simulink model "SistemaGrua_Planta_ModeloCompleto"  (R2020b)
settings: Solver=ode45  StartTime=0.0  StopTime=10  FixedStep=1e-3  RelTol=1e-3
values from neighbouring files (symbols this model uses):
  bcx = 1e6    (= 1000000)    [Valores_1.m]    (also in valoresPlanta.m; valoresPlanta_29_9_24.m; valoresPlanta_V3.m; valoresPlanta_v4.m)
  bcy = 1e7    (= 10000000)    [Valores_1.m]    (also in valoresPlanta.m; valoresPlanta_29_9_24.m; valoresPlanta_V3.m; valoresPlanta_v4.m)
  beq = bt+(btd+btm*it^2)/rtd^2    (= 21697.2)    [Valores.m]    (also in Valores_1.m; valoresPlanta_29_9_24.m; valoresPlanta_v4.m)
  bh_eq = bhm*ih^2+bhd    (= 8720)    [Valores.m]    (also in Valores_1.m; valoresPlanta.m; valoresPlanta_29_9_24.m; valoresPlanta_V3.m)
  bhb = 1e8    (= 100000000)    [Valores.m]    (also in Valores_1.m; valoresPlanta.m; valoresPlanta_29_9_24.m; valoresPlanta_V3.m)
  bhEb = 2.2e9    (= 2200000000)    [Valores.m]    (also in Valores_1.m; valoresPlanta.m; valoresPlanta_29_9_24.m; valoresPlanta_V3.m)
  bt = 90.0    (= 90)    [Valores.m]    (also in Valores_1.m; valoresPlanta.m; valoresPlanta_29_9_24.m; valoresPlanta_V3.m)
  btm = 6.0    (= 6)    [Valores.m]    (also in Valores_1.m; valoresPlanta.m; valoresPlanta_29_9_24.m; valoresPlanta_V3.m)
  btw = 3.0e3    (= 3000)    [Valores.m]    (also in Valores_1.m; valoresPlanta.m; valoresPlanta_29_9_24.m; valoresPlanta_V3.m)
  bwu = 150    [Valores.m]    (also in Valores_1.m; valoresPlanta.m; valoresPlanta_29_9_24.m; valoresPlanta_V3.m)
  g = 9.80665    [Valores.m]    (also in Valores_1.m; valoresPlanta.m; valoresPlanta_29_9_24.m; valoresPlanta_V3.m)
  ih = 22    [Valores.m]    (also in Valores_1.m; valoresPlanta.m; valoresPlanta_29_9_24.m; valoresPlanta_V3.m)
  it = 30    [Valores.m]    (also in Valores_1.m; valoresPlanta.m; valoresPlanta_29_9_24.m; valoresPlanta_V3.m)
  Jh_eq = Jhm_hb*ih^2+Jhd_hEb    (= 18320)    [Valores.m]    (also in Valores_1.m; valoresPlanta.m; valoresPlanta_29_9_24.m; valoresPlanta_V3.m)
  Jtm_tb = 7.0    (= 7)    [Valores.m]    (also in Valores_1.m; valoresPlanta.m; valoresPlanta_29_9_24.m; valoresPlanta_V3.m)
  kcy = 1.8e9    (= 1800000000)    [Valores_1.m]    (also in valoresPlanta.m; valoresPlanta_29_9_24.m; valoresPlanta_V3.m; valoresPlanta_v4.m)
  KDh = Jeq2 * w_posh^3    (= -12245.4404091)    [Valores.m]    (also in Valores_1.m = Jeq2 * w_posh; valoresPlanta.m = Jeq2 * w_posh; valoresPlanta_29_9_24.m = Jh_eq * n * w_posh; valoresPlanta_V3.m = Jeq2 * w_posh)
  KDt = Meq2 * w_post^3    (= -4728.86946035)    [Valores.m]    (also in Valores_1.m = Meq2 * w_post; valoresPlanta.m = Meq2 * w_post; valoresPlanta_29_9_24.m = 10127; valoresPlanta_V3.m = Meq2 * w_post)
  KIh = Jeq2 * w_posh^2    (= 2572.66592082)    [Valores.m]    (also in Valores_1.m = Jeq2 * w_posh^3; valoresPlanta.m = Jeq2 * w_posh^3; valoresPlanta_29_9_24.m = Jh_eq * w_posh^3; valoresPlanta_V3.m = Jeq2 * w_posh^3)
  KIt = Meq2 * w_post^2    (= 1307.690244)    [Valores.m]    (also in Valores_1.m = Meq2 * w_post^3; valoresPlanta.m = Meq2 * w_post^3; valoresPlanta_29_9_24.m = 6809.6; valoresPlanta_V3.m = Meq2 * w_post^3)
  KPh = Jeq2 * w_posh    (= -540.495867769)    [Valores.m]    (also in Valores_1.m = Jeq2 * w_posh^2; valoresPlanta.m = Jeq2 * w_posh^2; valoresPlanta_29_9_24.m = Jh_eq * n * w_posh^2; valoresPlanta_V3.m = Jeq2 * w_posh^2)
  KPt = Meq2 * w_post    (= -361.62)    [Valores.m]    (also in Valores_1.m = Meq2 * w_post^2; valoresPlanta.m = Meq2 * w_post^2; valoresPlanta_29_9_24.m = 14123; valoresPlanta_V3.m = Meq2 * w_post^2)
  Ktw = 4.8e5    (= 480000)    [Valores.m]    (also in Valores_1.m; valoresPlanta.m; valoresPlanta_29_9_24.m; valoresPlanta_V3.m)
  kwu = 2.36e8    (= 236000000)    [Valores.m]    (also in Valores_1.m; valoresPlanta.m; valoresPlanta_29_9_24.m; valoresPlanta_V3.m)
  Mc_max = 5e4    (= 50000)    [Valores.m]    (also in Valores_1.m; valoresPlanta.m; valoresPlanta_29_9_24.m; valoresPlanta_V3.m)
  Mc_min = 2e3    (= 2000)    [Valores.m]    (also in Valores_1.m; valoresPlanta.m; valoresPlanta_29_9_24.m; valoresPlanta_V3.m)
  Meq = Mt+(it^2*Jtm_tb+Jtd)/rtd^2    (= 60000)    [Valores.m]    (also in Valores_1.m; valoresPlanta_29_9_24.m; valoresPlanta_v4.m)
  Ms = 1.5e4    (= 15000)    [Valores.m]    (also in Valores_1.m; valoresPlanta.m; valoresPlanta_29_9_24.m; valoresPlanta_V3.m)
  Mt = 30000    [Valores.m]    (also in Valores_1.m; valoresPlanta.m; valoresPlanta_29_9_24.m; valoresPlanta_V3.m)
  rhd = 0.75    [Valores.m]    (also in Valores_1.m; valoresPlanta.m; valoresPlanta_29_9_24.m; valoresPlanta_V3.m)
  rtd = 0.5    [Valores.m]    (also in Valores_1.m; valoresPlanta.m; valoresPlanta_29_9_24.m; valoresPlanta_V3.m)
  tau_tm = 1e-3    (= 0.001)    [Valores.m]    (also in Valores_1.m; valoresPlanta.m; valoresPlanta_29_9_24.m; valoresPlanta_V3.m)
  tauhm = 1e-3    (= 0.001)    [Valores.m]    (also in Valores_1.m)
  Thb_Max = 5e4    (= 50000)    [Valores.m]    (also in Valores_1.m; valoresPlanta.m; valoresPlanta_29_9_24.m; valoresPlanta_V3.m)
  ThEb_Max = 1.1e6    (= 1100000)    [Valores.m]    (also in Valores_1.m; valoresPlanta.m; valoresPlanta_29_9_24.m; valoresPlanta_V3.m)
  Thm_Max = 2e4    (= 20000)    [Valores.m]    (also in Valores_1.m; valoresPlanta.m; valoresPlanta_29_9_24.m; valoresPlanta_V3.m)
  Ttb_Max = 5e3    (= 5000)    [Valores.m]    (also in Valores_1.m; valoresPlanta.m; valoresPlanta_29_9_24.m; valoresPlanta_V3.m)
  Ttm_Max = 3e3    (= 3000)    [Valores.m]    (also in Valores_1.m; valoresPlanta.m; valoresPlanta_29_9_24.m = 4000; valoresPlanta_V3.m)
  Yt0 = 45    [Valores.m]    (also in Valores_1.m; valoresPlanta.m; valoresPlanta_29_9_24.m; valoresPlanta_V3.m)
undefined symbols (not defined in the file or in its folder): DiscIntNeverNeededParam, sigbuilder_block
libraries: simulink x1, simulink_extras x1
settings Model: Creator=Matias  LastModifiedBy=agustin

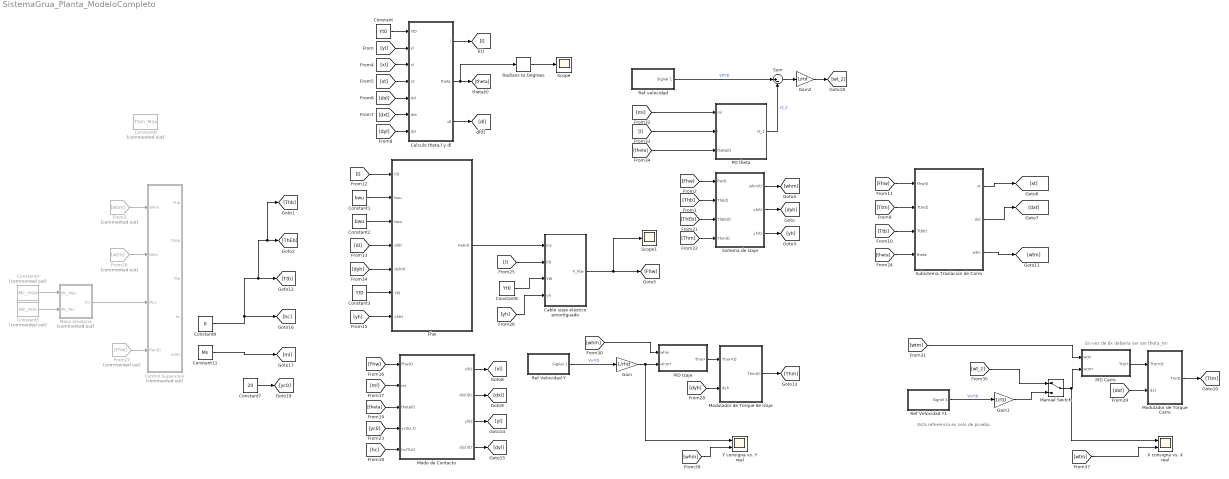
== system SistemaGrua_Planta_ModeloCompleto ==
  note: Esta referencia es solo de prueba
  note: En vez de dx debería ser ser theta_tm
  Cable izaje elástico amortiguado : Subsystem
  Calculo theta,l y dl : Subsystem
  Constant : Constant  Value=Yt0
  Constant1 : Constant  Value=kwu
  Constant11 : Constant  Value=Ms
  Constant2 : Constant  Value=bwu
  Constant3 : Constant  Value=Yt0
  Constant4 : Constant  Commented=on  Value=Mc_max
  Constant5 : Constant  Commented=on  Value=Mc_min
  Constant6 : Constant  Commented=on  Value=Thm_Max
  Constant7 : Constant  Value=20
  Constant8 : Constant  Value=Yt0
  Constant9 : Constant  Value=0
  Control Supervisor : Subsystem  Commented=on
  Fhw : Subsystem
  From20 : From  Commented=on  GotoTag=wtm
  From27 : From  Commented=on  GotoTag=Fhw
  From3 : From  Commented=on  GotoTag=whm
  Gain : Gain  Gain=1/rhd
  Gain1 : Gain  Gain=1/rtd
  Gain2 : Gain  Gain=1/rtd
  Manual Switch : ManualSwitch
  Masa aleatoria : MATLAB Function  Commented=on  TreatAsAtomicUnit=on
  Modo de Contacto : Subsystem
  Modulador de Torque Carro : Subsystem
  Modulador de Torque de Izaje : Subsystem
  PD theta : Subsystem
  PID Carro : Subsystem
  PID Izaje : Subsystem
  Radians to Degrees : simulink_extras/Transformations/Radians to Degrees
  Ref Velocidad Y : Subsystem  Tag=STV Subsys  LoadFcn=sigbuilder_block('load');  StartFcn=sigbuilder_block('start');  StopFcn=sigbuilder_block('stop');  ClipboardFcn=sigbuilder_block('clipboard');  mask(Sigbuilder block){tuvar=[0:10]}
      mask help: Simulink:masks:SigbuilderBlock_MD
      mask init:
      | if ~strcmp(get_param(bdroot(gcbh),'SimulationStatus'),'stopped') tuvar = sigbuilder_block('maskInit'); end
      settings: CopyFcn=sigbuilder_block('copy');  DeleteFcn=sigbuilder_block('delete');  ModelCloseFcn=sigbuilder_block('modelClose');  PreSaveFcn=sigbuilder_block('preSave');  PauseFcn=sigbuilder_block('pause');  ContinueFcn=sigbuilder_block('continue');  NameChangeFcn=sigbuilder_block('namechange');  OpenFcn=sigbuilder_block('open',[6 36 1012.5 476.25 ]);  CloseFcn=sigbuilder_block('close');
      mask Display: plot(0, 0, 100, 100,[2, 2, 32, 32, 2], [68, 8, 8, 68, 68],[32, 2], [38, 38], [32, 19, 2],[53, 60, 44], [32, 17, 17, 2],[16, 16, 31, 31]);txt = getActiveGroup(gcbh);text(2, 100, txt,'verticalAlignment', 'top');
  Ref Velocidad Y1 : Subsystem  Tag=STV Subsys  LoadFcn=sigbuilder_block('load');  StartFcn=sigbuilder_block('start');  StopFcn=sigbuilder_block('stop');  ClipboardFcn=sigbuilder_block('clipboard');  mask(Sigbuilder block){tuvar=[0:10]}
      mask help: Simulink:masks:SigbuilderBlock_MD
      mask init:
      | if ~strcmp(get_param(bdroot(gcbh),'SimulationStatus'),'stopped') tuvar = sigbuilder_block('maskInit'); end
      settings: CopyFcn=sigbuilder_block('copy');  DeleteFcn=sigbuilder_block('delete');  ModelCloseFcn=sigbuilder_block('modelClose');  PreSaveFcn=sigbuilder_block('preSave');  PauseFcn=sigbuilder_block('pause');  ContinueFcn=sigbuilder_block('continue');  NameChangeFcn=sigbuilder_block('namechange');  OpenFcn=sigbuilder_block('open',[6 30 1012.5 447.75 ]);  CloseFcn=sigbuilder_block('close');
      mask Display: plot(0, 0, 100, 100,[2, 2, 32, 32, 2], [68, 8, 8, 68, 68],[32, 2], [38, 38], [32, 19, 2],[53, 60, 44], [32, 17, 17, 2],[16, 16, 31, 31]);txt = getActiveGroup(gcbh);text(2, 100, txt,'verticalAlignment', 'top');
  Ref velocidad : Subsystem  Tag=STV Subsys  LoadFcn=sigbuilder_block('load');  StartFcn=sigbuilder_block('start');  StopFcn=sigbuilder_block('stop');  ClipboardFcn=sigbuilder_block('clipboard');  mask(Sigbuilder block){tuvar=[0:10]}
      mask help: Simulink:masks:SigbuilderBlock_MD
      mask init:
      | if ~strcmp(get_param(bdroot(gcbh),'SimulationStatus'),'stopped') tuvar = sigbuilder_block('maskInit'); end
      settings: CopyFcn=sigbuilder_block('copy');  DeleteFcn=sigbuilder_block('delete');  ModelCloseFcn=sigbuilder_block('modelClose');  PreSaveFcn=sigbuilder_block('preSave');  PauseFcn=sigbuilder_block('pause');  ContinueFcn=sigbuilder_block('continue');  NameChangeFcn=sigbuilder_block('namechange');  OpenFcn=sigbuilder_block('open',[6 36 1012.5 476.25 ]);  CloseFcn=sigbuilder_block('close');
      mask Display: plot(0, 0, 100, 100,[2, 2, 32, 32, 2], [68, 8, 8, 68, 68],[32, 2], [38, 38], [32, 19, 2],[53, 60, 44], [32, 17, 17, 2],[16, 16, 31, 31]);txt = getActiveGroup(gcbh);text(2, 100, txt,'verticalAlignment', 'top');
  Scope : Scope
  Scope1 : Scope
  Sistema de Izaje : Subsystem
  Subsitema Traslación de Carro : Subsystem
  Sum : Sum  Inputs=|+-
  X consigna vs. X real : Scope  NumInputPorts=2
  Y consigna vs. Y real : Scope  NumInputPorts=2
  wires:
  From3/1 -> Control Supervisor/1(Whm)
  [Thb] -> Sistema de Izaje/2(Thb(t))
  [Fhw] -> Sistema de Izaje/1(Fw(t))
  Calculo theta,l y dl/1(l) -> [l]
  Calculo theta,l y dl/2(theta) -> [theta], Radians to Degrees/1
  Constant/1 -> Calculo theta,l y dl/1(Yt0)
  [xt] -> Calculo theta,l y dl/4(xt)
  [xl] -> Calculo theta,l y dl/3(xl)
  [yl] -> Calculo theta,l y dl/2(yl)
  Calculo theta,l y dl/3(dl) -> [dl]
  [dyl] -> Calculo theta,l y dl/7(dyl)
  [dxt] -> Calculo theta,l y dl/6(dxt)
  [dxl] -> Calculo theta,l y dl/5(dxl)
  [yh] -> Fhw/7(yh(t))
  [dyh] -> Fhw/5(dyh(t))
  [dl] -> Fhw/4(dl(t))
  [l] -> Fhw/1(l(t))
  Constant1/1 -> Fhw/2(kwu)
  Constant2/1 -> Fhw/3(bwu)
  [Ttb] -> Subsitema Traslación de Carro/3(Ttb(t))
  [Fhw] -> Subsitema Traslación de Carro/1(Fhw(t))
  [Ttm] -> Subsitema Traslación de Carro/2(Ttm(t))
  Subsitema Traslación de Carro/1(xt) -> [xt]
  Subsitema Traslación de Carro/2(dxt) -> [dxt]
  Modulador de Torque Carro/1(Tm(t)) -> [Ttm]
  Subsitema Traslación de Carro/3(wtm) -> [wtm]
  From20/1 -> Control Supervisor/2(Wtm)
  Modulador de Torque de Izaje/1(Thm(t)) -> [Thm]
  Sistema de Izaje/1(whm(t)) -> [whm]
  Sistema de Izaje/2(vh(t)) -> [dyh]
  Sistema de Izaje/3(yh(t)) -> [yh]
  [ThEb] -> Sistema de Izaje/3(ThEb(t))
  [Thm] -> Sistema de Izaje/4(Thm(t))
  Constant3/1 -> Fhw/6(Yt0)
  Constant5/1 -> Masa aleatoria/2(Mc_Min)
  Constant4/1 -> Masa aleatoria/1(Mc_Max)
  Masa aleatoria/1(ml) -> Control Supervisor/3(Mcx)
  [theta] -> Subsitema Traslación de Carro/4(theta)
  [yc0] -> Modo de Contacto/4(yc0(x,t))
  Modo de Contacto/2(d(xl)(t)) -> [dxl]
  Modo de Contacto/1(xl(t)) -> [xl]
  [hc] -> Modo de Contacto/5(hc(TLK))
  Modo de Contacto/4(d(yl)(t)) -> [dyl]
  [theta] -> Modo de Contacto/3(theta(t))
  Modo de Contacto/3(yl(t)) -> [yl]
  [ml] -> Modo de Contacto/2(ml)
  [Fhw] -> Modo de Contacto/1(Fhw(t))
  Fhw/1(Fwh(t)) -> Cable izaje elástico amortiguado/1(In1)
  [l] -> Cable izaje elástico amortiguado/2(l(t))
  Constant8/1 -> Cable izaje elástico amortiguado/3(Yt0)
  [yh] -> Cable izaje elástico amortiguado/4(yh)
  From27/1 -> Control Supervisor/4(Fwh(t))
  [dyh] -> Modulador de Torque de Izaje/2(dyh)
  [dxt] -> Modulador de Torque Carro/2(dxt)
  PID Carro/1(Ttm*) -> Modulador de Torque Carro/1(Ttm*(t)')
  PID Izaje/1(Thm*) -> Modulador de Torque de Izaje/1(Thm*(t)')
  [wtm] -> PID Carro/1(wtm)
  [whm] -> PID Izaje/1(whm)
  Ref Velocidad Y/1(Signal 1) -> Gain/1  "Vy*(t)"
  [wt_2] -> Manual Switch/1
  [whm] -> Y consigna vs. Y real/2
  [wtm] -> X consigna vs. X real/2
  Ref velocidad/1(Signal 1) -> Sum/1  "Vt*(t)"
  Sum/1 -> Gain2/1
  Gain2/1 -> [wt_2]
  Manual Switch/1 -> X consigna vs. X real/1, PID Carro/2(wtm*)
  Ref Velocidad Y1/1(Signal 1) -> Gain1/1  "Vx*(t)"
  Gain1/1 -> Manual Switch/2
  Gain/1 -> Y consigna vs. Y real/1, PID Izaje/2(whm*)
  [theta] -> PD theta/3(theta(t))
  [l] -> PD theta/2(l)
  PD theta/1(xt_2) -> Sum/2  "xt_2"
  [ml] -> PD theta/1(ml)
  Cable izaje elástico amortiguado/1(F_htw) -> Scope1/1, [Fhw]
  Constant7/1 -> [yc0]
  Constant11/1 -> [ml]
  Constant9/1 -> [Thb], [ThEb], [Ttb], [hc]
  Radians to Degrees/1 -> Scope/1

== system SistemaGrua_Planta_ModeloCompleto/Cable izaje elástico amortiguado ==
  note: l_h
  In1 : Inport
  l(t) : Inport  Port=2
  Yt0 : Inport  Port=3
  yh : Inport  Port=4
  Constant9 : Constant  Value=0
  Relational Operator : RelationalOperator  OutDataTypeStr=boolean  RndMeth=Simplest
  Sum : Sum  Inputs=|++
  Switch1 : Switch  Criteria=u2 > Threshold
  F_htw : Outport
  wires:
  l(t)/1 -> Relational Operator/1
  Sum/1 -> Relational Operator/2
  In1/1 -> Switch1/1
  Yt0/1 -> Sum/1
  Constant9/1 -> Switch1/3
  Relational Operator/1 -> Switch1/2
  yh/1 -> Sum/2
  Switch1/1 -> F_htw/1

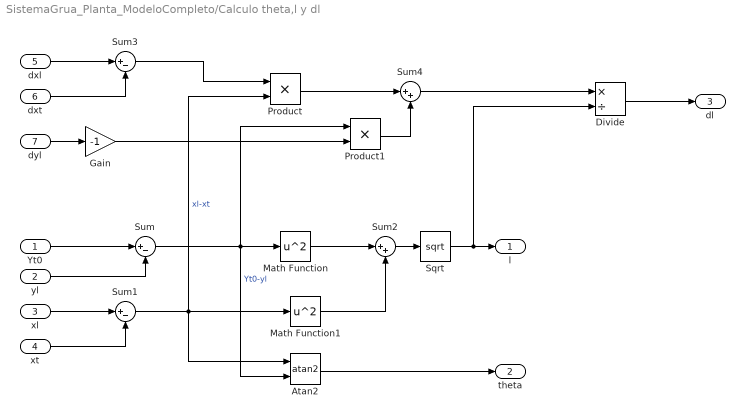
== system SistemaGrua_Planta_ModeloCompleto/Calculo theta,l y dl ==
  Yt0 : Inport
  yl : Inport  Port=2
  xl : Inport  Port=3
  xt : Inport  Port=4
  dxl : Inport  Port=5
  dxt : Inport  Port=6
  dyl : Inport  Port=7
  Atan2 : Trigonometry  Operator=atan2
  Divide : Product  Inputs=*/
  Gain : Gain  Gain=-1
  Math Function : Math  Operator=square  SaturateOnIntegerOverflow=on
  Math Function1 : Math  Operator=square  SaturateOnIntegerOverflow=on
  Product : Product
  Product1 : Product
  Sqrt : Sqrt  SaturateOnIntegerOverflow=on
  Sum : Sum  Inputs=|+-
  Sum1 : Sum  Inputs=|+-
  Sum2 : Sum  Inputs=|++
  Sum3 : Sum  Inputs=|+-
  Sum4 : Sum  Inputs=|++
  l : Outport
  theta : Outport  Port=2
  dl : Outport  Port=3
  wires:
  Yt0/1 -> Sum/1
  yl/1 -> Sum/2
  xl/1 -> Sum1/1
  xt/1 -> Sum1/2
  Atan2/1 -> theta/1
  Sum1/1 -> Product/2, Math Function1/1, Atan2/1  "xl-xt"
  Sum/1 -> Product1/1, Atan2/2, Math Function/1  "Yt0-yl"
  Math Function/1 -> Sum2/1
  Math Function1/1 -> Sum2/2
  Sum2/1 -> Sqrt/1
  Sqrt/1 -> Divide/2, l/1
  dxl/1 -> Sum3/1
  dxt/1 -> Sum3/2
  Sum3/1 -> Product/1
  dyl/1 -> Gain/1
  Gain/1 -> Product1/2
  Product/1 -> Sum4/1
  Product1/1 -> Sum4/2
  Sum4/1 -> Divide/1
  Divide/1 -> dl/1

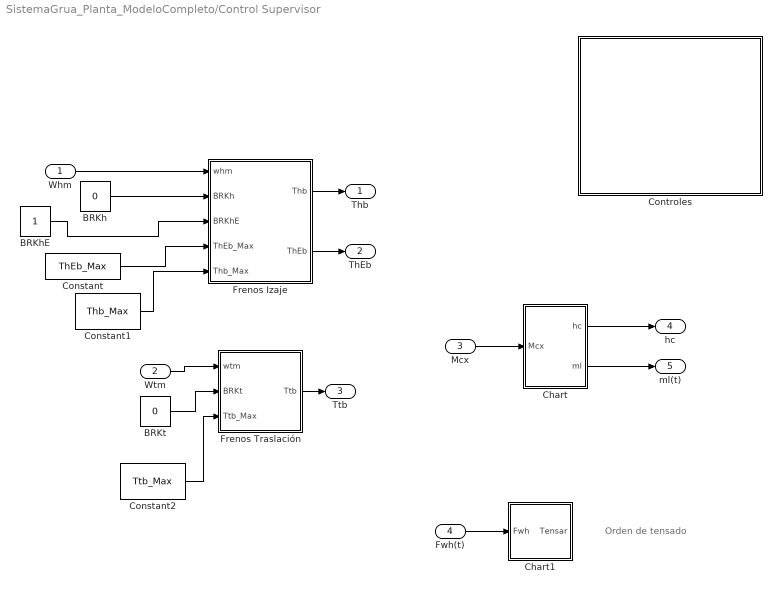
== system SistemaGrua_Planta_ModeloCompleto/Control Supervisor ==
  note: Orden de tensado
  Whm : Inport
  Wtm : Inport  Port=2
  Mcx : Inport  Port=3
  Fwh(t) : Inport  Port=4
  BRKh : Constant  Value=0
  BRKhE : Constant
  BRKt : Constant  Value=0
  Chart : Stateflow chart  TreatAsAtomicUnit=on
  Chart1 : Stateflow chart  TreatAsAtomicUnit=on
  Constant : Constant  Value=ThEb_Max
  Constant1 : Constant  Value=Thb_Max
  Constant2 : Constant  Value=Ttb_Max
  Controles : Subsystem
  "Frenos Izaje " : Stateflow chart  TreatAsAtomicUnit=on
  Frenos Traslación : Stateflow chart  TreatAsAtomicUnit=on
  Thb : Outport
  ThEb : Outport  Port=2
  Ttb : Outport  Port=3
  hc : Outport  Port=4
  ml(t) : Outport  Port=5
  wires:
  "Frenos Izaje "/1(Thb) -> Thb/1
  BRKh/1 -> "Frenos Izaje "/2(BRKh)
  Whm/1 -> "Frenos Izaje "/1(whm)
  BRKhE/1 -> "Frenos Izaje "/3(BRKhE)
  "Frenos Izaje "/2(ThEb) -> ThEb/1
  Wtm/1 -> Frenos Traslación/1(wtm)
  Frenos Traslación/1(Ttb) -> Ttb/1
  BRKt/1 -> Frenos Traslación/2(BRKt)
  Chart/2(ml) -> ml(t)/1
  Chart/1(hc) -> hc/1
  Mcx/1 -> Chart/1(Mcx)
  Fwh(t)/1 -> Chart1/1(Fwh)
  Constant/1 -> "Frenos Izaje "/4(ThEb_Max)
  Constant1/1 -> "Frenos Izaje "/5(Thb_Max)
  Constant2/1 -> Frenos Traslación/3(Ttb_Max)

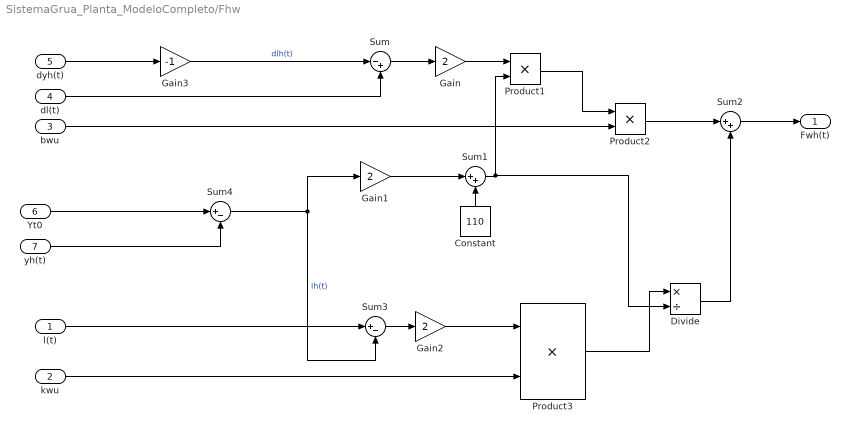
== system SistemaGrua_Planta_ModeloCompleto/Fhw ==
  l(t) : Inport
  kwu : Inport  Port=2
  bwu : Inport  Port=3
  dl(t) : Inport  Port=4
  dyh(t) : Inport  Port=5
  Yt0 : Inport  Port=6
  yh(t) : Inport  Port=7
  Constant : Constant  Value=110
  Divide : Product  Inputs=*/
  Gain : Gain  Gain=2
  Gain1 : Gain  Gain=2
  Gain2 : Gain  Gain=2
  Gain3 : Gain  Gain=-1
  Product1 : Product
  Product2 : Product
  Product3 : Product
  Sum : Sum  Inputs=|-+
  Sum1 : Sum  Inputs=|++
  Sum2 : Sum  Inputs=|++
  Sum3 : Sum  Inputs=|+-
  Sum4 : Sum  Inputs=|+-
  Fwh(t) : Outport
  wires:
  dl(t)/1 -> Sum/2
  Sum/1 -> Gain/1
  Gain1/1 -> Sum1/1
  Sum4/1 -> Sum3/2, Gain1/1  "lh(t)"
  l(t)/1 -> Sum3/1
  Constant/1 -> Sum1/2
  Gain/1 -> Product1/1
  Sum1/1 -> Product1/2, Divide/2
  Product1/1 -> Product2/1
  bwu/1 -> Product2/2
  Product2/1 -> Sum2/1
  Sum3/1 -> Gain2/1
  Gain2/1 -> Product3/1
  kwu/1 -> Product3/2
  Product3/1 -> Divide/1
  Divide/1 -> Sum2/2
  Sum2/1 -> Fwh(t)/1
  dyh(t)/1 -> Gain3/1
  Gain3/1 -> Sum/1  "dlh(t)"
  Yt0/1 -> Sum4/1
  yh(t)/1 -> Sum4/2

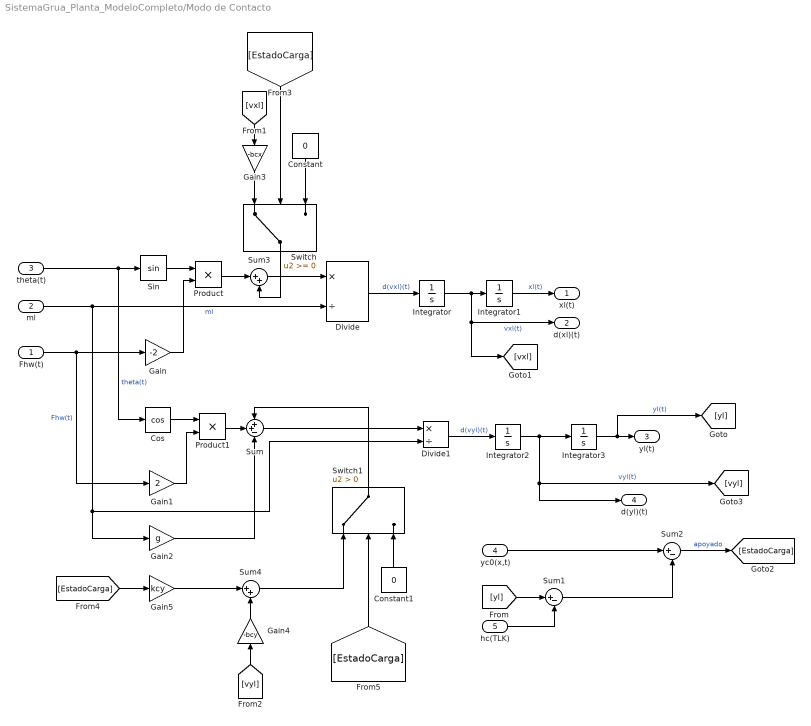
== system SistemaGrua_Planta_ModeloCompleto/Modo de Contacto ==
  Fhw(t) : Inport
  ml : Inport  Port=2
  theta(t) : Inport  Port=3
  yc0(x,t) : Inport  Port=4
  hc(TLK) : Inport  Port=5
  Constant : Constant  Value=0
  Constant1 : Constant  Value=0
  Cos : Trigonometry  Operator=cos
  Divide : Product  Inputs=*/
  Divide1 : Product  Inputs=*/
  Gain : Gain  Gain=-2
  Gain1 : Gain  Gain=2
  Gain2 : Gain  Gain=g
  Gain3 : Gain  Gain=-bcx
  Gain4 : Gain  Gain=-bcy
  Gain5 : Gain  Gain=kcy
  Integrator{,1..3} (4 alike) : Integrator
  Product : Product
  Product1 : Product
  Sin : Trigonometry
  Sum : Sum  Inputs=++-
  Sum1 : Sum  Inputs=|+-
  Sum2 : Sum  Inputs=|+-
  Sum3 : Sum  Inputs=|++
  Sum4 : Sum  Inputs=|++
  Switch : Switch
  Switch1 : Switch  Criteria=u2 > Threshold
  xl(t) : Outport
  d(xl)(t) : Outport  Port=2
  yl(t) : Outport  Port=3
  d(yl)(t) : Outport  Port=4
  wires:
  theta(t)/1 -> Sin/1, Cos/1  "theta(t)"
  Fhw(t)/1 -> Gain/1, Gain1/1  "Fhw(t)"
  Sin/1 -> Product/1
  Gain/1 -> Product/2
  ml/1 -> Gain2/1, Divide1/2, Divide/2  "ml"
  Divide/1 -> Integrator/1  "d(vxl)(t)"
  Integrator1/1 -> xl(t)/1  "xl(t)"
  Cos/1 -> Product1/1
  Gain1/1 -> Product1/2
  Divide1/1 -> Integrator2/1  "d(vyl)(t)"
  Integrator3/1 -> [yl], yl(t)/1  "yl(t)"
  Integrator/1 -> Integrator1/1, [vxl], d(xl)(t)/1  "vxl(t)"
  Integrator2/1 -> Integrator3/1, [vyl], d(yl)(t)/1  "vyl(t)"
  hc(TLK)/1 -> Sum1/2
  [yl] -> Sum1/1
  yc0(x,t)/1 -> Sum2/1
  Sum1/1 -> Sum2/2
  Product/1 -> Sum3/1
  Sum3/1 -> Divide/1
  Switch/1 -> Sum3/2
  [vxl] -> Gain3/1
  Sum/1 -> Divide1/1
  Product1/1 -> Sum/2
  Gain2/1 -> Sum/3
  [vyl] -> Gain4/1
  Switch1/1 -> Sum/1
  Sum2/1 -> [EstadoCarga]  "apoyado"
  [EstadoCarga] -> Switch/2
  Gain4/1 -> Sum4/2
  [EstadoCarga] -> Gain5/1
  Gain5/1 -> Sum4/1
  [EstadoCarga] -> Switch1/2
  Constant/1 -> Switch/3
  Gain3/1 -> Switch/1
  Constant1/1 -> Switch1/3
  Sum4/1 -> Switch1/1

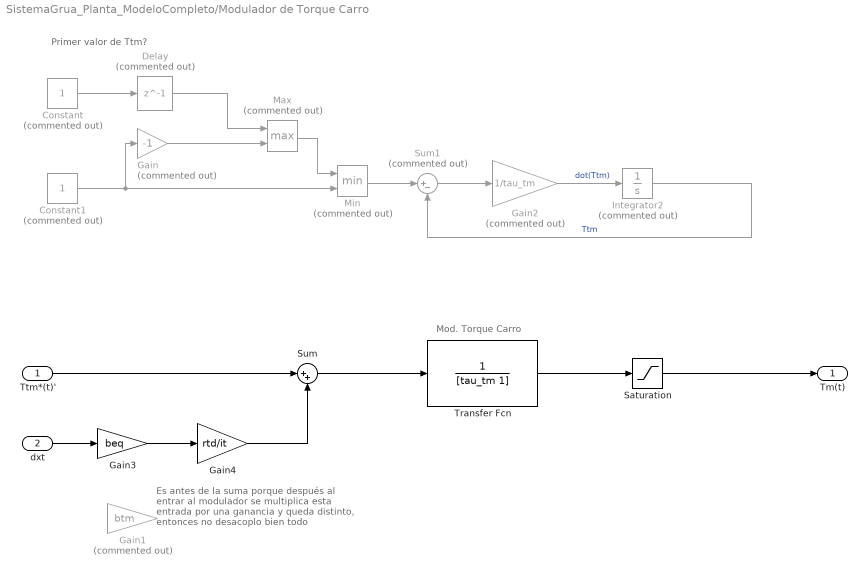
== system SistemaGrua_Planta_ModeloCompleto/Modulador de Torque Carro ==
  note: Es antes de la suma porque después
      | al entrar al modulador se multiplica
      | esta entrada por una ganancia y queda
      | distinto, entonces no desacoplo bien todo
  note: Primer valor de Ttm?
  note: Mod. Torque Carro
  Ttm*(t)' : Inport
  dxt : Inport  Port=2
  Constant : Constant  Commented=on
  Constant1 : Constant  Commented=on
  Delay : Delay  Commented=on  DelayLength=1  InitialCondition=0
  Gain : Gain  Commented=on  Gain=-1
  Gain1 : Gain  Commented=on  Gain=btm
  Gain2 : Gain  Commented=on  Gain=1/tau_tm
  Gain3 : Gain  Gain=beq
  Gain4 : Gain  Gain=rtd/it
  Integrator2 : Integrator  Commented=on
  Max : MinMax  Commented=on  Function=max  Inputs=2
  Min : MinMax  Commented=on  Inputs=2
  Saturation : Saturate  UpperLimit=Ttm_Max  LowerLimit=-Ttm_Max
  Sum : Sum  Inputs=|++
  Sum1 : Sum  Commented=on  Inputs=|+-
  Transfer Fcn : TransferFcn  Denominator=[tau_tm 1]
  Tm(t) : Outport
  wires:
  Integrator2/1 -> Sum1/2  "Ttm"
  Sum1/1 -> Gain2/1
  Gain2/1 -> Integrator2/1  "dot(Ttm)"
  Constant/1 -> Delay/1
  Gain/1 -> Max/2
  Delay/1 -> Max/1
  Max/1 -> Min/1
  Min/1 -> Sum1/1
  Constant1/1 -> Gain/1, Min/2
  Gain3/1 -> Gain4/1
  Ttm*(t)'/1 -> Sum/1
  Sum/1 -> Transfer Fcn/1
  dxt/1 -> Gain3/1
  Transfer Fcn/1 -> Saturation/1
  Gain4/1 -> Sum/2
  Saturation/1 -> Tm(t)/1

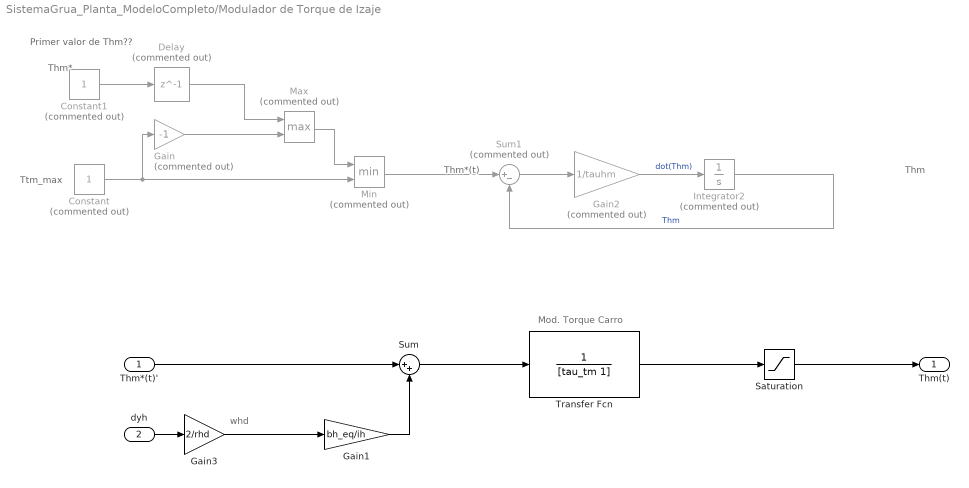
== system SistemaGrua_Planta_ModeloCompleto/Modulador de Torque de Izaje ==
  note: whd
  note: Mod. Torque Carro
  note: Thm
  note: Thm*
  note: Ttm_max
  note: Primer valor de Thm??
  note: Thm*(t)
  Thm*(t)' : Inport
  dyh : Inport  Port=2
  Constant : Constant  Commented=on
  Constant1 : Constant  Commented=on
  Delay : Delay  Commented=on  DelayLength=1  InitialCondition=0
  Gain : Gain  Commented=on  Gain=-1
  Gain1 : Gain  Gain=bh_eq/ih
  Gain2 : Gain  Commented=on  Gain=1/tauhm
  Gain3 : Gain  Gain=2/rhd
  Integrator2 : Integrator  Commented=on
  Max : MinMax  Commented=on  Function=max  Inputs=2
  Min : MinMax  Commented=on  Inputs=2
  Saturation : Saturate  UpperLimit=Thm_Max  LowerLimit=-Thm_Max
  Sum : Sum  Inputs=|++
  Sum1 : Sum  Commented=on  Inputs=|+-
  Transfer Fcn : TransferFcn  Denominator=[tau_tm 1]
  Thm(t) : Outport
  wires:
  Integrator2/1 -> Sum1/2  "Thm"
  Constant1/1 -> Delay/1
  Sum1/1 -> Gain2/1
  Gain2/1 -> Integrator2/1  "dot(Thm)"
  Constant/1 -> Gain/1, Min/2
  Gain/1 -> Max/2
  Delay/1 -> Max/1
  Max/1 -> Min/1
  Min/1 -> Sum1/1
  Transfer Fcn/1 -> Saturation/1
  Sum/1 -> Transfer Fcn/1
  Thm*(t)'/1 -> Sum/1
  Gain3/1 -> Gain1/1
  dyh/1 -> Gain3/1
  Gain1/1 -> Sum/2
  Saturation/1 -> Thm(t)/1

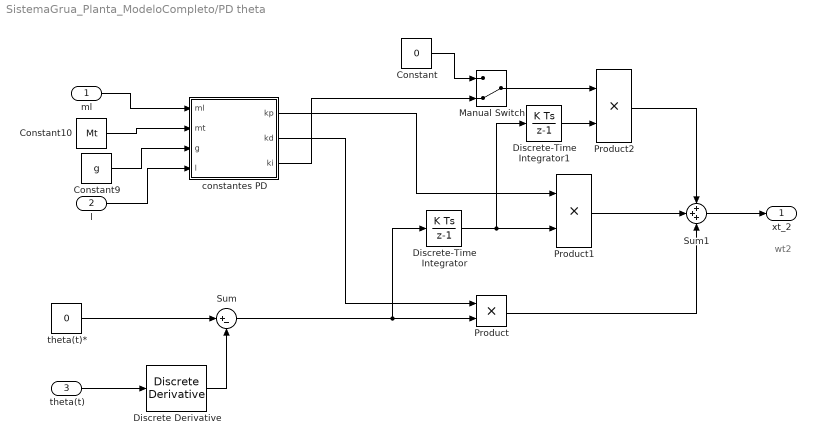
== system SistemaGrua_Planta_ModeloCompleto/PD theta ==
  note: wt2
  ml : Inport
  l : Inport  Port=2
  theta(t) : Inport  Port=3
  Constant : Constant  Value=0
  Constant10 : Constant  Value=Mt
  Constant9 : Constant  Value=g
  Discrete Derivative : simulink/Quick Insert/Discrete/Discrete Derivative  gainval=1.0  ICPrevScaledInput=0.0  OutMin=[]  OutMax=[]  OutDataType=fixdt(1, 16)  OutScaling=2^-10  DoSatur=off
      settings: SourceProductBaseCode=SL
  Discrete-Time Integrator : DiscreteIntegrator  SampleTime=-1  ICPrevOutput=DiscIntNeverNeededParam  ICPrevScaledInput=DiscIntNeverNeededParam
  Discrete-Time Integrator1 : DiscreteIntegrator  SampleTime=-1  ICPrevOutput=DiscIntNeverNeededParam  ICPrevScaledInput=DiscIntNeverNeededParam
  Manual Switch : ManualSwitch  CurrentSetting=0
  Product : Product
  Product1 : Product
  Product2 : Product
  Sum : Sum  Inputs=|+-
  Sum1 : Sum  Inputs=+++
  "constantes PD " : MATLAB Function  TreatAsAtomicUnit=on
  theta(t)* : Constant  Value=0
  xt_2 : Outport
  wires:
  l/1 -> "constantes PD "/4(l)
  Product/1 -> Sum1/3
  Constant10/1 -> "constantes PD "/2(mt)
  ml/1 -> "constantes PD "/1(ml)
  Sum/1 -> Product/2, Discrete-Time Integrator/1
  theta(t)/1 -> Discrete Derivative/1
  Product1/1 -> Sum1/2
  Constant9/1 -> "constantes PD "/3(g)
  theta(t)*/1 -> Sum/1
  Sum1/1 -> xt_2/1
  "constantes PD "/2(kd) -> Product/1
  Discrete-Time Integrator/1 -> Discrete-Time Integrator1/1, Product1/2
  "constantes PD "/1(kp) -> Product1/1
  Discrete Derivative/1 -> Sum/2
  Discrete-Time Integrator1/1 -> Product2/2
  "constantes PD "/3(ki) -> Manual Switch/2
  Product2/1 -> Sum1/1
  Manual Switch/1 -> Product2/1
  Constant/1 -> Manual Switch/1

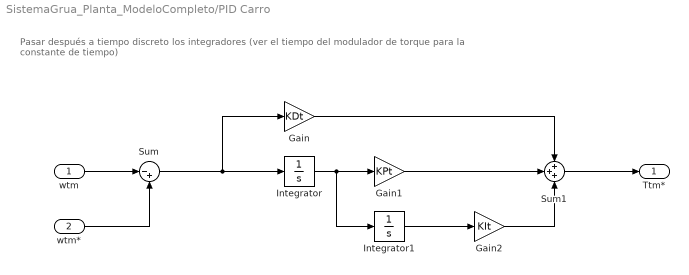
== system SistemaGrua_Planta_ModeloCompleto/PID Carro ==
  note: Pasar después a tiempo discreto los integradores (ver el tiempo del modulador de torque para la constante de tiempo)
  wtm : Inport
  wtm* : Inport  Port=2
  Gain : Gain  Gain=KDt
  Gain1 : Gain  Gain=KPt
  Gain2 : Gain  Gain=KIt
  Integrator : Integrator
  Integrator1 : Integrator
  Sum : Sum  Inputs=|-+
  Sum1 : Sum  Inputs=+++
  Ttm* : Outport
  wires:
  wtm/1 -> Sum/1
  wtm*/1 -> Sum/2
  Sum/1 -> Integrator/1, Gain/1
  Integrator/1 -> Integrator1/1, Gain1/1
  Integrator1/1 -> Gain2/1
  Gain2/1 -> Sum1/3
  Gain1/1 -> Sum1/2
  Gain/1 -> Sum1/1
  Sum1/1 -> Ttm*/1

== system SistemaGrua_Planta_ModeloCompleto/PID Izaje ==
  note: Pasar después a tiempo discreto los integradores (ver el tiempo del modulador de torque para la constante de tiempo)
  whm : Inport
  whm* : Inport  Port=2
  Gain : Gain  Gain=KDh
  Gain1 : Gain  Gain=KPh
  Gain2 : Gain  Gain=KIh
  Integrator : Integrator
  Integrator1 : Integrator
  Sum : Sum  Inputs=|-+
  Sum1 : Sum  Inputs=+++
  Thm* : Outport
  wires:
  whm/1 -> Sum/1
  whm*/1 -> Sum/2
  Sum/1 -> Integrator/1, Gain/1
  Integrator/1 -> Integrator1/1, Gain1/1
  Integrator1/1 -> Gain2/1
  Gain2/1 -> Sum1/3
  Gain1/1 -> Sum1/2
  Gain/1 -> Sum1/1
  Sum1/1 -> Thm*/1

== system SistemaGrua_Planta_ModeloCompleto/Ref Velocidad Y ==
  Demux : Demux  Tag=STV Demux  Outputs=1
      settings: DisplayOption=none
  FromWs : FromWorkspace  Tag=STV FromWs  VariableName=tuvar
      SigBuilderData=|
      | common.afterFinalStr = 'Extrapolate'
      | common.sampleTime = 0
      | dataSet.timeRange = [0 10]
      | dataSet.name = 'Group 1'
      | sbobj.Groups.Name = 'Group 1'
      | sbobj.Groups.Signals.Name = 'Signal 1'
      | sbobj.Groups.Signals.XData = [0 4 6 10]
      | sbobj.Groups.Signals.YData = [0 2 2 0]
  Signal 1 : Outport  Tag=STV Outport
  wires:
  Demux/1 -> Signal 1/1
  FromWs/1 -> Demux/1

== system SistemaGrua_Planta_ModeloCompleto/Ref Velocidad Y1 ==
  Demux : Demux  Tag=STV Demux  Outputs=1
      settings: DisplayOption=none
  FromWs : FromWorkspace  Tag=STV FromWs  VariableName=tuvar
      SigBuilderData=|
      | common.afterFinalStr = 'Extrapolate'
      | common.sampleTime = 0
      | dataSet.timeRange = [0 10]
      | dataSet.name = 'Group 1'
      | sbobj.Groups.Name = 'Group 1'
      | sbobj.Groups.Signals.Name = 'Signal 1'
      | sbobj.Groups.Signals.XData = [0 4 6 10]
      | sbobj.Groups.Signals.YData = [0 20 20 0]
  Signal 1 : Outport  Tag=STV Outport
  wires:
  Demux/1 -> Signal 1/1
  FromWs/1 -> Demux/1

== system SistemaGrua_Planta_ModeloCompleto/Ref velocidad ==
  Demux : Demux  Tag=STV Demux  Outputs=1
      settings: DisplayOption=none
  FromWs : FromWorkspace  Tag=STV FromWs  VariableName=tuvar
      SigBuilderData=|
      | common.afterFinalStr = 'Extrapolate'
      | common.sampleTime = 0
      | dataSet.timeRange = [0 10]
      | dataSet.name = 'Group 1'
      | sbobj.Groups.Name = 'Group 1'
      | sbobj.Groups.Signals.Name = 'Signal 1'
      | sbobj.Groups.Signals.XData = [0 4 6 10]
      | sbobj.Groups.Signals.YData = [0 2 2 0]
  Signal 1 : Outport  Tag=STV Outport
  wires:
  Demux/1 -> Signal 1/1
  FromWs/1 -> Demux/1

== system SistemaGrua_Planta_ModeloCompleto/Sistema de Izaje ==
  Fw(t) : Inport
  Thb(t) : Inport  Port=2
  ThEb(t) : Inport  Port=3
  Thm(t) : Inport  Port=4
  Sistema Fisico Izaje : Subsystem
  whm(t) : Outport
  vh(t) : Outport  Port=2
  yh(t) : Outport  Port=3
  wires:
  Fw(t)/1 -> Sistema Fisico Izaje/1(Fw(t))
  Thb(t)/1 -> Sistema Fisico Izaje/2(Thb(t))
  Thm(t)/1 -> Sistema Fisico Izaje/3(Thm(t))
  Sistema Fisico Izaje/1(whm(t)) -> whm(t)/1
  Sistema Fisico Izaje/2(vh(t)) -> vh(t)/1
  Sistema Fisico Izaje/3(yh(t)) -> yh(t)/1
  ThEb(t)/1 -> Sistema Fisico Izaje/4(ThEb(t))

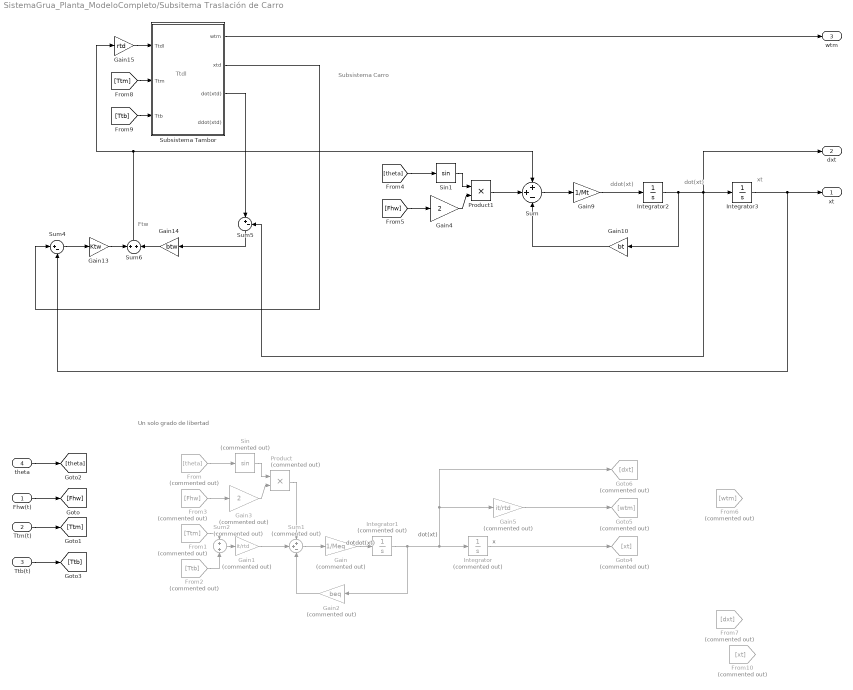
== system SistemaGrua_Planta_ModeloCompleto/Subsitema Traslación de Carro ==
  note: Ftw
  note: Ttdl
  note: Subsistema Carro
  note: dot(xt)
  note: ddot(xt)
  note: Un solo grado de libertad
  note: x
  note: dot(xt)
  note: dotdot(xt)
  note: xt
  Fhw(t) : Inport
  Ttm(t) : Inport  Port=2
  Ttb(t) : Inport  Port=3
  theta : Inport  Port=4
  From : From  Commented=on  GotoTag=theta
  From1 : From  Commented=on  GotoTag=Ttm
  From10 : From  Commented=on  GotoTag=xt
  From2 : From  Commented=on  GotoTag=Ttb
  From3 : From  Commented=on  GotoTag=Fhw
  From6 : From  Commented=on  GotoTag=wtm
  From7 : From  Commented=on  GotoTag=dxt
  Gain : Gain  Commented=on  Gain=1/Meq
  Gain1 : Gain  Commented=on  Gain=it/rtd
  Gain10 : Gain  Gain=bt
  Gain13 : Gain  Gain=Ktw
  Gain14 : Gain  Gain=btw
  Gain15 : Gain  Gain=rtd
  Gain2 : Gain  Commented=on  Gain=beq
  Gain3 : Gain  Commented=on  Gain=2
  Gain4 : Gain  Gain=2
  Gain5 : Gain  Commented=on  Gain=it/rtd
  Gain9 : Gain  Gain=1/Mt
  Goto4 : Goto  Commented=on  GotoTag=xt
  Goto5 : Goto  Commented=on  GotoTag=wtm
  Goto6 : Goto  Commented=on  GotoTag=dxt
  Integrator : Integrator  Commented=on
  Integrator1 : Integrator  Commented=on
  Integrator2 : Integrator
  Integrator3 : Integrator
  Product : Product  Commented=on
  Product1 : Product
  Sin : Trigonometry  Commented=on
  Sin1 : Trigonometry
  Subsistema Tambor : Subsystem
  Sum : Sum  Inputs=++-
  Sum1 : Sum  Commented=on  Inputs=++-
  Sum2 : Sum  Commented=on
  Sum4 : Sum  Inputs=|+-
  Sum5 : Sum  Inputs=|+-
  Sum6 : Sum
  xt : Outport
  dxt : Outport  Port=2
  wtm : Outport  Port=3
  wires:
  Sin/1 -> Product/1
  Gain1/1 -> Sum1/2
  Integrator1/1 -> Gain2/1, Goto6/1, Gain5/1, Integrator/1
  Sum2/1 -> Gain1/1
  Gain3/1 -> Product/2
  Gain2/1 -> Sum1/3
  Gain/1 -> Integrator1/1
  Sum1/1 -> Gain/1
  Product/1 -> Sum1/1
  Fhw(t)/1 -> [Fhw]
  Ttb(t)/1 -> [Ttb]
  Ttm(t)/1 -> [Ttm]
  Gain5/1 -> Goto5/1
  Integrator/1 -> Goto4/1
  theta/1 -> [theta]
  From/1 -> Sin/1
  From3/1 -> Gain3/1
  From1/1 -> Sum2/1
  From2/1 -> Sum2/2
  Gain4/1 -> Product1/2
  Sin1/1 -> Product1/1
  [Fhw] -> Gain4/1
  [theta] -> Sin1/1
  Product1/1 -> Sum/2
  Sum6/1 -> Sum/1, Gain15/1
  Subsistema Tambor/3(dot(xtd)) -> Sum5/1
  Sum/1 -> Gain9/1
  Gain9/1 -> Integrator2/1
  Gain10/1 -> Sum/3
  Subsistema Tambor/2(xtd) -> Sum4/1
  Sum4/1 -> Gain13/1
  Sum5/1 -> Gain14/1
  Gain14/1 -> Sum6/2
  Gain13/1 -> Sum6/1
  [Ttb] -> Subsistema Tambor/3(Ttb)
  [Ttm] -> Subsistema Tambor/2(Ttm)
  Gain15/1 -> Subsistema Tambor/1(Ttdl)
  Integrator3/1 -> xt/1, Sum4/2
  Integrator2/1 -> Gain10/1, dxt/1, Sum5/2, Integrator3/1
  Subsistema Tambor/1(wtm) -> wtm/1

== system SistemaGrua_Planta_ModeloCompleto/Control Supervisor/Controles ==
  Lamp : LampBlock
  Lamp1 : LampBlock
  Lamp2 : LampBlock
  Rocker Switch : RockerSwitchBlock
      settings: Values={{'Off', 'On'}, [0 1]}
  Rocker Switch1 : RockerSwitchBlock
      settings: Values={{'Off', 'On'}, [0 1]}
  Rocker Switch2 : RockerSwitchBlock
      settings: Values={{'Off', 'On'}, [0 1]}

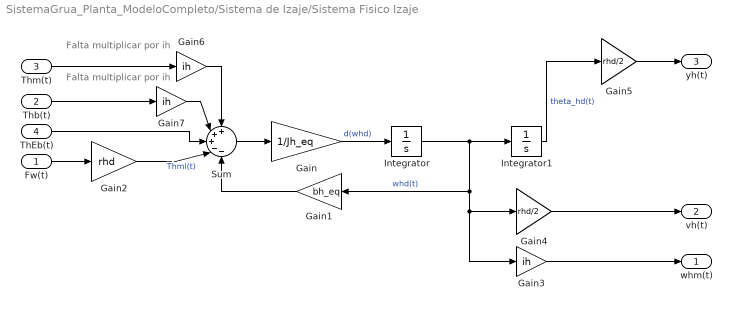
== system SistemaGrua_Planta_ModeloCompleto/Sistema de Izaje/Sistema Fisico Izaje ==
  note: Falta multiplicar por ih
  note: Falta multiplicar por ih
  Fw(t) : Inport
  Thb(t) : Inport  Port=2
  Thm(t) : Inport  Port=3
  ThEb(t) : Inport  Port=4
  Gain : Gain  Gain=1/Jh_eq
  Gain1 : Gain  Gain=bh_eq
  Gain2 : Gain  Gain=rhd
  Gain3 : Gain  Gain=ih
  Gain4 : Gain  Gain=rhd/2
  Gain5 : Gain  Gain=rhd/2
  Gain6 : Gain  Gain=ih
  Gain7 : Gain  Gain=ih
  Integrator : Integrator
  Integrator1 : Integrator
  Sum : Sum  Inputs=+++--
  whm(t) : Outport
  vh(t) : Outport  Port=2
  yh(t) : Outport  Port=3
  wires:
  Gain/1 -> Integrator/1  "d(whd)"
  Sum/1 -> Gain/1
  Integrator/1 -> Gain3/1, Gain4/1, Gain1/1, Integrator1/1  "whd(t)"
  Fw(t)/1 -> Gain2/1
  Thb(t)/1 -> Gain7/1
  Thm(t)/1 -> Gain6/1
  Gain1/1 -> Sum/5
  Gain2/1 -> Sum/4  "Thml(t)"
  ThEb(t)/1 -> Sum/3
  Gain3/1 -> whm(t)/1
  Gain4/1 -> vh(t)/1
  Integrator1/1 -> Gain5/1  "theta_hd(t)"
  Gain5/1 -> yh(t)/1
  Gain6/1 -> Sum/1
  Gain7/1 -> Sum/2

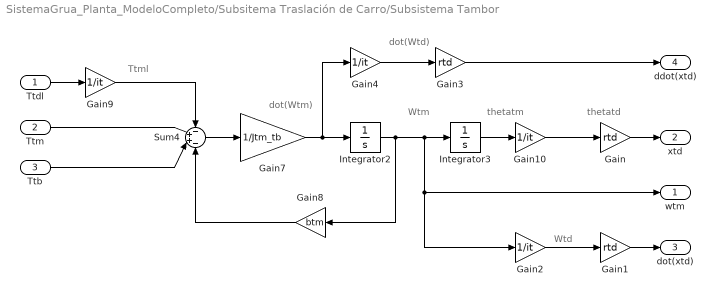
== system SistemaGrua_Planta_ModeloCompleto/Subsitema Traslación de Carro/Subsistema Tambor ==
  note: dot(Wtm)
  note: Ttml
  note: Wtm
  note: thetatm
  note: thetatd
  note: Wtd
  note: dot(Wtd)
  Ttdl : Inport
  Ttm : Inport  Port=2
  Ttb : Inport  Port=3
  Gain : Gain  Gain=rtd
  Gain1 : Gain  Gain=rtd
  Gain{2,4,9..10} (4 alike) : Gain  Gain=1/it
  Gain3 : Gain  Gain=rtd
  Gain7 : Gain  Gain=1/Jtm_tb
  Gain8 : Gain  Gain=btm
  Integrator2 : Integrator
  Integrator3 : Integrator
  Sum4 : Sum  Inputs=-++-
  wtm : Outport
  xtd : Outport  Port=2
  dot(xtd) : Outport  Port=3
  ddot(xtd) : Outport  Port=4
  wires:
  Ttdl/1 -> Gain9/1
  Integrator2/1 -> wtm/1, Gain2/1, Integrator3/1, Gain8/1
  Ttb/1 -> Sum4/3
  Gain8/1 -> Sum4/4
  Ttm/1 -> Sum4/2
  Gain7/1 -> Gain4/1, Integrator2/1
  Gain9/1 -> Sum4/1
  Sum4/1 -> Gain7/1
  Gain10/1 -> Gain/1
  Gain/1 -> xtd/1
  Integrator3/1 -> Gain10/1
  Gain1/1 -> dot(xtd)/1
  Gain2/1 -> Gain1/1
  Gain4/1 -> Gain3/1
  Gain3/1 -> ddot(xtd)/1

== stateflow chart SistemaGrua_Planta_ModeloCompleto/Control Supervisor/Chart1 ==
  (default) -> (junction 8) : % Deteccion de cable flojo
  (junction 8) -> (junction 9) [order 1] : [Fwh>0]
  (junction 8) -> (junction 10) [order 2] : {Tensar=1}
  (junction 9) -> (junction 11) : {Tensar=0;}
  (junction 11) -> (junction 10)
  (junction 10) -> (junction 12)
  data: Fwh input; Tensar output =0

== matlab function SistemaGrua_Planta_ModeloCompleto/PD theta/constantes PD  ==
  data: ml input; kp output; mt input; g input; l input; kd output; ki output
function [kp,kd,ki] = fcn(ml,mt,g,l)
    xita=0.7;
    wn=(mt*g/((mt+ml)*l))^(1/2);
    kd=-(mt*g/((mt+ml)*(wn^(3))));
    kp=kd*(2*xita*wn-wn)+l;
    ki=wn^2*(1-xita)*kd;

== stateflow chart SistemaGrua_Planta_ModeloCompleto/Control Supervisor/Frenos Traslación ==
  state FrenosOperacion
    state BRKt_off
      during:
      Ttb=-btb*wtm;
      Ttb=min(Ttb_Max,Ttb);
    state BRKt_on
      during:
      Ttb=0;
    (default) -> BRKt_off
    BRKt_off -> BRKt_on : [BRKt==1 ]
    BRKt_on -> BRKt_off : [BRKt==0]
  data: Ttb output; wtm input; btb parameter; BRKt input; Ttb_Max input

== stateflow chart SistemaGrua_Planta_ModeloCompleto/Control Supervisor/Chart ==
  state TLK_OFF
    during:
    hc=0;
    ml=Ms;
  state TLK_ON
    during:
    hc=2.5;
    ml=Ms+Mcx;
  (default) -> TLK_OFF
  TLK_OFF -> TLK_ON : [Mcx>0]
  TLK_ON -> TLK_OFF : [Mcx<=0]
  data: Mcx input; hc output; ml output; Ms parameter

== stateflow chart SistemaGrua_Planta_ModeloCompleto/Control Supervisor/Frenos Izaje  ==
  state FrenosOperacion
    state BRKh_off
      during:
      Thb=-bhb*whm;
      Thb=min(Thb_Max,Thb);
    state BRKh_on
      during:
      Thb=0;
    (default) -> BRKh_off
    BRKh_off -> BRKh_on [order 1] : [BRKh==1 && BRKhE==1]
    BRKh_on -> BRKh_off [order 1] : [BRKh==0 && BRKhE==1]
  state FrenosEmergencia
    state BRKhE_off
      during:
      ThEb=-bhEb*whm;
      ThEb=min(ThEb_Max,ThEb);
    state BRKhE_on
      during:
      ThEb=0;
    (default) -> BRKhE_off
    BRKhE_off -> BRKhE_on : [BRKhE==1]
    BRKhE_on -> BRKhE_off [order 1] : [BRKhE==0]
  BRKh_on -> FrenosEmergencia [order 2] : [BRKhE==0]
  BRKh_off -> FrenosEmergencia [order 2] : [BRKhE==0]
  BRKhE_on -> FrenosOperacion [order 2] : [BRKhE==1]
  (default) -> FrenosEmergencia
  data: Thb output; whm input; bhb parameter; BRKh input; ThEb output; bhEb parameter; BRKhE input; ThEb_Max input; Thb_Max input

== matlab function SistemaGrua_Planta_ModeloCompleto/Masa aleatoria ==
  data: Mc_Max input; ml output; Mc_Min input
function ml = fcn(Mc_Max, Mc_Min)
%Cambiar los valores de tiempo a criterio
tic;
while (1)
    tic;
    t = randi([5,8],1);
    elapsed_time = toc;
    %elapsed_time = end_time - start_time;
    while elapsed_time < t
        ml = Mc_Min + (Mc_Max - Mc_Min)*rand(1); %genero numero aleatorio
        %disp(ml);
        pause(1);
        elapsed_time = elapsed_time + toc;
    end
    %fprintf("Masa excedida")
    ml = Mc_Max + 0.01 * randi([1,15],1) * Mc_Max;   %genero aleatorio con sobrecarga (hasta 15% mas)
    %disp(ml);
    pause(1);   %Pausa de 5 segundos
    elapsed_time = 0;
end
